simulink subsystem "Matlab_Mission_Manager"  (R2025b)
settings: Solver=VariableStepAuto  StartTime=0.0  StopTime=10.0  RelTol=1e-3
libraries: ros2lib x2
settings Model: Creator=kjhaydon  LastModifiedBy=kjhaydon

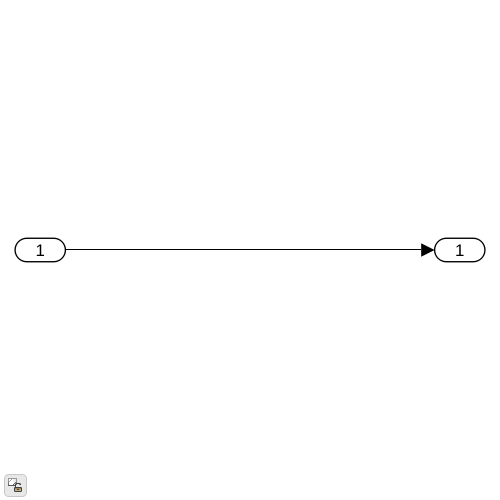
[thumbnail: Simulink's stored preview of the top-level diagram]
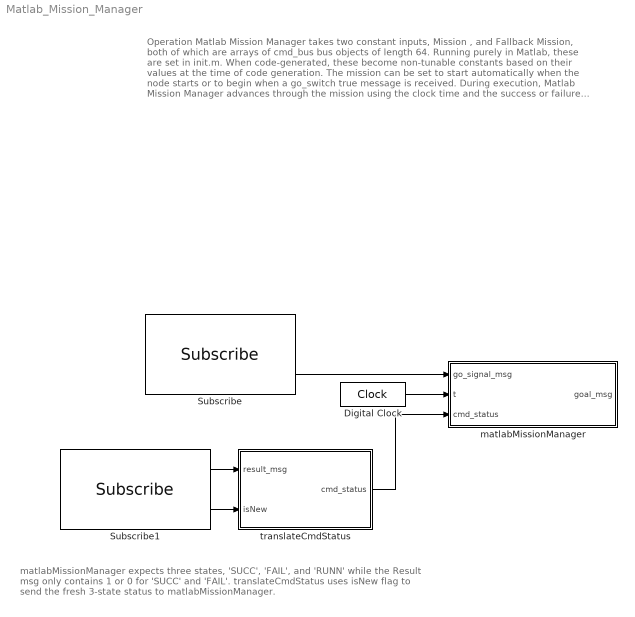
== system Matlab_Mission_Manager ==
  note: matlabMissionManager expects three states, 'SUCC', 'FAIL', and 'RUNN' while
      | the Result msg only contains 1 or 0 for 'SUCC' and 'FAIL'. translateCmdStatus uses
      | isNew flag to send the fresh 3-state status to matlabMissionManager.
  note: Operation
      | Matlab Mission Manager takes two constant inputs, Mission , and Fallback Mission, both of which are arrays of cmd_bus bus objects of length 64. Running purely in Matlab, these are set in init.m. When code-generated, these become non-tunable constants based on their values at the time of code generation.
      |
      | The mission can be set to start automatically when the node starts or to begin when a go_switch true message is received.
      |
      | During execution, Matlab Mission Manager advances through the mission using the clock time and the success or failure status to advance the mission. If a failure occurs, the mission manager switches to the Fallback Mission. If the mission ends, Matlab Mission Manager continues to hold whatever the final command of the mission was.
  Digital Clock : DigitalClock
  Subscribe : ros2lib/Subscribe  topicSource=Specify your own  topic=/go_signal  messageType=std_msgs/Bool  sampleTime=dt_control  QOSHistory=Keep last  QOSDepth=10  QOSReliability=Reliable  QOSDurability=Volatile  QOSDeadline=Inf  QOSLifespan=Inf  QOSLiveliness=Automatic  QOSLeaseDuration=Inf  QOSAvoidROSNamespaceConventions=off
  Subscribe1 : ros2lib/Subscribe  topicSource=Specify your own  topic=/cmd_result  messageType=custom_interfaces/Result  sampleTime=dt_control  QOSHistory=Keep last  QOSDepth=10  QOSReliability=Reliable  QOSDurability=Volatile  QOSDeadline=Inf  QOSLifespan=Inf  QOSLiveliness=Automatic  QOSLeaseDuration=Inf  QOSAvoidROSNamespaceConventions=off
  matlabMissionManager : MATLAB Function  TreatAsAtomicUnit=on
  translateCmdStatus : MATLAB Function  TreatAsAtomicUnit=on
  wires:
  Subscribe/2 -> matlabMissionManager/1(go_signal_msg)
  Digital Clock/1 -> matlabMissionManager/2(t)
  Subscribe1/1 -> translateCmdStatus/1(result_msg)
  Subscribe1/2 -> translateCmdStatus/2(isNew)
  translateCmdStatus/1(cmd_status) -> matlabMissionManager/3(cmd_status)

== matlab function Matlab_Mission_Manager/matlabMissionManager ==
  data: go_signal_msg input Bus: SL_Bus_std_msgs_Bool; goal_msg output Bus: SL_Bus_custom_interfaces_Goal; mission parameter Bus: cmd_name size=max_commands_in_mission; t input; cmd_status input
function goal_msg = fcn(go_signal_msg, mission, t, cmd_status)
%{
Note the variable Type settings in Function -> Edit Data.
go_signal_msg: [1x1 SL_Bus_std_msgs_Bool]
    .data [1x1 bool]
mission: [max_commands_in_mission x 1 cmd_bus]
cmd_status: [1x4 int8]


goal_msg: [SL_Bus_custom_interfaces_Goal]
    



%}

y = matlabMissionManager(go_signal_msg, mission, t, cmd_status);

== matlab function Matlab_Mission_Manager/translateCmdStatus ==
  data: result_msg input Bus: SL_Bus_custom_interfaces_Result; isNew input; cmd_status output
function cmd_status = fcn(result_msg, isNew)

cmd_status = translateCmdStatus(result_msg, isNew);
